simulink model "SOGI_PLL"  (R2018a)
settings: Solver=FixedStepAuto  StartTime=0.0  StopTime=2  FixedStep=1e-4  RelTol=1e-3
undefined symbols (not defined in the file or in its folder): DiscIntNeverNeededParam
settings Model: Creator=donghao  LastModifiedBy=donghao
settings SolverCC: AlgebraicLoopSolver=LineSearch

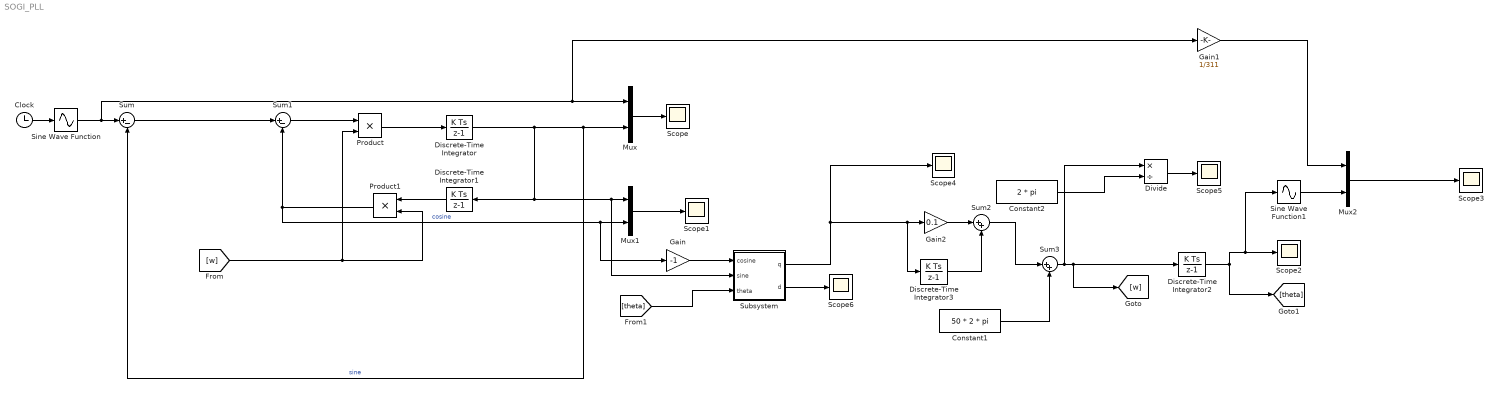
== system SOGI_PLL ==
  Clock : Clock
  Constant1 : Constant  Value=50 * 2 * pi
  Constant2 : Constant  Value=2 * pi
  Discrete-Time Integrator{,1..3} (4 alike) : DiscreteIntegrator  gainval=1  SampleTime=1e-4  ICPrevOutput=DiscIntNeverNeededParam  ICPrevScaledInput=DiscIntNeverNeededParam
  Divide : Product  Inputs=*/
  Gain : Gain  Gain=-1
  Gain1 : Gain  Gain=1/311
  Gain2 : Gain  Gain=0.1
  Mux : Mux  Inputs=2
  Mux1 : Mux  Inputs=2
  Mux2 : Mux  Inputs=2
  Product : Product
  Product1 : Product
  Scope{,1..6} (7 alike) : Scope
  Sine Wave Function : Sin  TimeSource=Use external signal  Amplitude=311  Frequency=50 * 2 * pi  Phase=1.5  SampleTime=0
  Sine Wave Function1 : Sin  TimeSource=Use external signal  SampleTime=0
  Subsystem : Subsystem
  Sum : Sum  Inputs=|+-
  Sum1 : Sum  Inputs=|+-
  Sum2 : Sum  Inputs=|++
  Sum3 : Sum  Inputs=|++
  wires:
  Clock/1 -> Sine Wave Function/1
  Sum/1 -> Sum1/1
  Sum1/1 -> Product/1
  Product/1 -> Discrete-Time Integrator/1
  Discrete-Time Integrator/1 -> Subsystem/2(sine), Mux1/1, Discrete-Time Integrator1/1, Mux/2, Sum/2  "sine"
  Discrete-Time Integrator1/1 -> Product1/1
  Product1/1 -> Gain/1, Mux1/2, Sum1/2  "cosine"
  [w] -> Product1/2, Product/2
  Mux/1 -> Scope/1
  Mux1/1 -> Scope1/1
  Sum2/1 -> Sum3/1
  Constant1/1 -> Sum3/2
  Sum3/1 -> Divide/1, Discrete-Time Integrator2/1, [w]
  Discrete-Time Integrator2/1 -> Sine Wave Function1/1, Scope2/1, [theta]
  Mux2/1 -> Scope3/1
  Sine Wave Function1/1 -> Mux2/2
  Sine Wave Function/1 -> Gain1/1, Mux/1, Sum/1
  [theta] -> Subsystem/3(theta)
  Divide/1 -> Scope5/1
  Constant2/1 -> Divide/2
  Subsystem/2(d) -> Scope6/1
  Gain1/1 -> Mux2/1
  Gain/1 -> Subsystem/1(cosine)
  Subsystem/1(q) -> Discrete-Time Integrator3/1, Gain2/1, Scope4/1
  Gain2/1 -> Sum2/1
  Discrete-Time Integrator3/1 -> Sum2/2

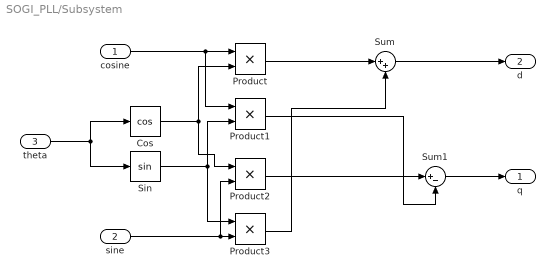
== system SOGI_PLL/Subsystem ==
  cosine : Inport
  sine : Inport  Port=2
  theta : Inport  Port=3
  Cos : Trigonometry  Operator=cos
  Product{,1..3} (4 alike) : Product
  Sin : Trigonometry
  Sum : Sum  Inputs=|++
  Sum1 : Sum  Inputs=|+-
  q : Outport
  d : Outport  Port=2
  wires:
  theta/1 -> Sin/1, Cos/1
  cosine/1 -> Product1/1, Product/1
  Cos/1 -> Product2/1, Product/2
  Sin/1 -> Product3/1, Product1/2
  sine/1 -> Product2/2, Product3/2
  Sum/1 -> d/1
  Product/1 -> Sum/1
  Product3/1 -> Sum/2
  Product2/1 -> Sum1/1
  Product1/1 -> Sum1/2
  Sum1/1 -> q/1
